simulink model "DriveModeSim"  (R2024b)
settings: Solver=VariableStepAuto  StartTime=0.0  StopTime=10.0  RelTol=1e-3
libraries: simulink x3, SignalEditorBlockLib x1
settings Model: Creator=carlo  LastModifiedBy=carlo

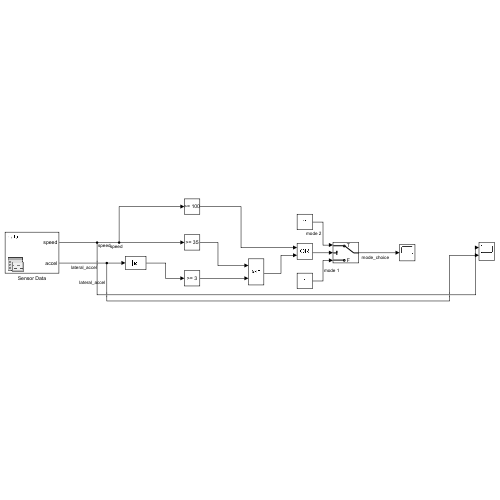
[thumbnail: Simulink's stored preview of the top-level diagram]
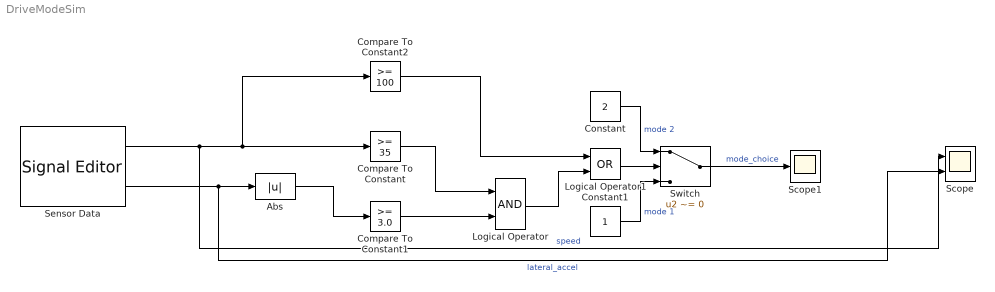
== system DriveModeSim ==
  Abs : Abs  SaturateOnIntegerOverflow=off
  Compare To Constant : simulink/Logic and Bit Operations/Compare To Constant  relop=>=  const=35  OutDataTypeStr=boolean
  Compare To Constant1 : simulink/Logic and Bit Operations/Compare To Constant  relop=>=  const=3.0  OutDataTypeStr=boolean
  Compare To Constant2 : simulink/Logic and Bit Operations/Compare To Constant  relop=>=  const=100  OutDataTypeStr=boolean
  Constant : Constant  Value=2
  Constant1 : Constant
  Logical Operator : Logic  AllPortsSameDT=off  OutDataTypeStr=boolean
  Logical Operator1 : Logic  Operator=OR  AllPortsSameDT=off  OutDataTypeStr=boolean
  Scope : Scope  NumInputPorts=2
  Scope1 : Scope
  Sensor Data : SignalEditorBlockLib/Signal Editor  FileName=signalData.mat  ActiveScenario=data  ActiveSignal=speed  IsBus=off  OutputBusObjectStr=Bus: BusObject  SampleTime=0  Interpolate=off  ZeroCross=off  OutputAfterFinalValue=Setting to zero  Unit=inherit  PreserveSignalName=on  ApplySigPropsToAllScenarios=on  ApplySigPropsToAllSignals=off
  Switch : Switch  Criteria=u2 ~= 0  Threshold=1  SaturateOnIntegerOverflow=off  InputSameDT=off
  wires:
  Compare To Constant1/1 -> Logical Operator/2
  Abs/1 -> Compare To Constant1/1
  Compare To Constant2/1 -> Logical Operator1/1
  Logical Operator/1 -> Logical Operator1/2
  Compare To Constant/1 -> Logical Operator/1
  Constant1/1 -> Switch/3  "mode 1"
  Sensor Data/2 -> Scope/2, Abs/1  "lateral_accel"
  Sensor Data/1 -> Scope/1, Compare To Constant2/1, Compare To Constant/1  "speed"
  Logical Operator1/1 -> Switch/2
  Constant/1 -> Switch/1  "mode 2"
  Switch/1 -> Scope1/1  "mode_choice"
